simulink model "IIR"  (R2016a)
settings: Solver=VariableStepAuto  StartTime=0.0  StopTime=10.0  RelTol=1e-3
libraries: dspsrcs4 x2
settings Model: Creator=joa-m  LastModifiedBy=joa-m

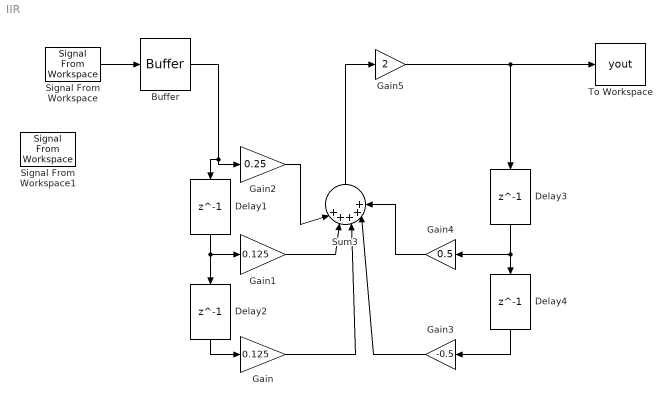
== system IIR ==
  Buffer : Buffer  N=1  TreatMby1Signals=One channel  OutputFrames=off
  Delay{1..4} (4 alike) : Delay  DelayLength=1  InputProcessing=Columns as channels (frame based)
  Gain : Gain  Gain=0.125
  Gain1 : Gain  Gain=0.125
  Gain2 : Gain  Gain=0.25
  Gain3 : Gain  Gain=-0.5
  Gain4 : Gain  Gain=0.5
  Gain5 : Gain  Gain=2
  Signal From Workspace : dspsrcs4/Signal From Workspace  X=[0.5,0]  Ts=1  nsamps=1  OutputAfterFinalValue=Setting to zero  ignoreOrWarnInputAndFrameLengths=off  OutputFrames=off
  Signal From Workspace1 : dspsrcs4/Signal From Workspace  X=[0.25,0.5,0,-0.25]  Ts=1  nsamps=1  OutputAfterFinalValue=Setting to zero  ignoreOrWarnInputAndFrameLengths=off  OutputFrames=off
  Sum3 : Sum  Inputs=|+++++
  To Workspace : ToWorkspace  VariableName=yout  SampleTime=-1
      settings: Save2DSignal=2-D array (concatenate along first dimension)
  wires:
  Signal From Workspace/1 -> Buffer/1
  Delay3/1 -> Gain4/1, Delay4/1
  Delay4/1 -> Gain3/1
  Delay2/1 -> Gain/1
  Delay1/1 -> Delay2/1, Gain1/1
  Buffer/1 -> Delay1/1, Gain2/1
  Gain3/1 -> Sum3/4
  Gain/1 -> Sum3/3
  Gain1/1 -> Sum3/2
  Gain2/1 -> Sum3/1
  Gain4/1 -> Sum3/5
  Sum3/1 -> Gain5/1
  Gain5/1 -> To Workspace/1, Delay3/1
